simulink model "MultirotorModel"  (R2021b)
settings: Solver=VariableStepAuto  StartTime=0.0  StopTime=200  FixedStep=0.005  RelTol=1e-3  EnableMultiTasking=on
undefined symbols (not defined in the file): Controller, decyear, DiscIntNeverNeededParam, DroneMass, Dz, Earth, Gravity, initialConditions, Iz, leapyear, Nz, Pz, startFlightTime, UAVSampleTime, Vehicle, WGS84
libraries: slpidlib x10, uavalgslib x6, aerolibtransform2 x4, simulink x2, sharedutil x2, aerolibconvert2 x2, aerolibatmos2 x1, aerolibgravity2 x1, shared6dof x1, aerolibasang x1, sensorinslib x1
(part 1 of 3)
settings Model: DataDictionary=uavPackageDeliveryDataDict.sldd  ModifiedByFormat=The MathWorks, Inc.  Creator=The MathWorks, Inc.  LastModifiedBy=The MathWorks, Inc.
settings SolverCC: AlgebraicLoopSolver=TrustRegion  AutoInsertRateTranBlk=on
settings DataIOCC: LimitDataPoints=on  SaveOutput=off  SaveTime=off  ReturnWorkspaceOutputs=off
settings OptimizationCC: LifeSpan=inf
settings DebuggingCC: ParameterPrecisionLossMsg=none  AllowSymbolicDim=off  SFUnexpectedBacktrackingDiag=warning  SFNoUnconditionalDefaultTransitionDiag=warning  SFExecutionAtInitializationDiag=none  SFMachineParentedDataDiag=warning  ArithmeticOperatorsInVariantConditions=warning
settings ModelReferenceCC: PropagateSignalLabelsOutOfModel=off
settings SFSimCC: SimUseLocalCustomCode=off  CustomCodeUndefinedFunction=UseInterfaceOnly
settings RTWCC: RTWUseLocalCustomCode=off
settings CodeAppCC: StateflowObjectComments=on
settings GRTTargetCC: TargetLangStandard=C89/C90 (ANSI)
settings ConfigComp: CovMetricSettings=dw  CovSaveCumulativeToWorkspaceVar=on  CovSaveSingleToWorkspaceVar=on  CovExternalEMLEnable=off

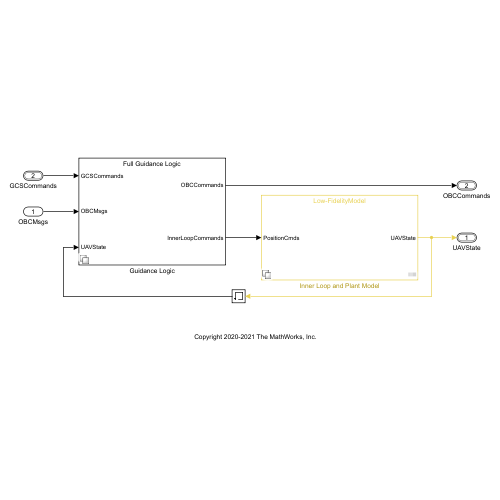
[thumbnail: Simulink's stored preview of the top-level diagram]
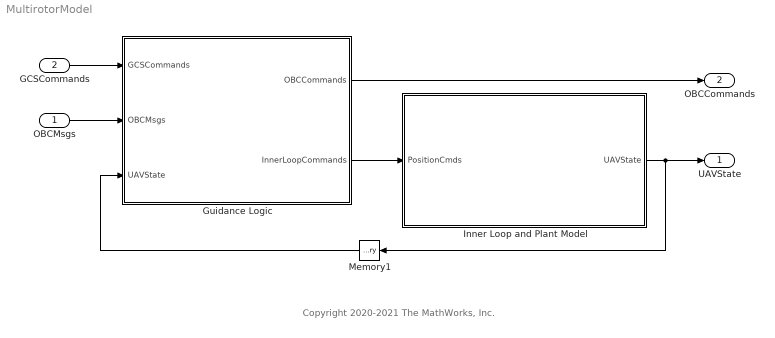
== system MultirotorModel ==
  note: Copyright 2020-2021 The MathWorks, Inc.
  OBCMsgs : Inport  OutDataTypeStr=single  PortDimensions=[1 1]  SampleTime=UAVSampleTime*4
  GCSCommands : Inport  Port=2  OutDataTypeStr=Bus: uavPathManagerBus  PortDimensions=42  SampleTime=UAVSampleTime*4  BusOutputAsStruct=on
  Guidance Logic : Subsystem  Variant=on
  Inner Loop and Plant Model : Subsystem  Variant=on
  Memory1 : Memory  InheritSampleTime=on
  UAVState : Outport  OutDataTypeStr=Bus: uavStateBus  BusOutputAsStruct=on
  OBCCommands : Outport  Port=2  OutDataTypeStr=Bus: uavPathManagerBus  PortDimensions=2  SampleTime=0.005  BusOutputAsStruct=on
  wires:
  GCSCommands/1 -> Guidance Logic/1(GCSCommands)
  OBCMsgs/1 -> Guidance Logic/2(OBCMsgs)
  Guidance Logic/2(InnerLoopCommands) -> Inner Loop and Plant Model/1(PositionCmds)
  Guidance Logic/1(OBCCommands) -> OBCCommands/1
  Inner Loop and Plant Model/1(UAVState) -> Memory1/1, UAVState/1
  Memory1/1 -> Guidance Logic/3(UAVState)

== system MultirotorModel/Guidance Logic ==
  GCSCommands : Inport
  OBCMsgs : Inport  Port=2
  UAVState : Inport  Port=3
  Full Guidance Logic : Subsystem  TreatAsAtomicUnit=on  SystemSampleTime=UAVSampleTime*4  VariantControl=guidanceType==1
  Obstacle Avoidance : Subsystem  TreatAsAtomicUnit=on  SystemSampleTime=0.005*4  VariantControl=guidanceType ==2
  OBCCommands : Outport  SampleTime=0.005  BusOutputAsStruct=on
  InnerLoopCommands : Outport  Port=2

== system MultirotorModel/Inner Loop and Plant Model ==
  PositionCmds : Inport
  High-FidelityModel : Subsystem  VariantControl=plantModelFi==1
  Low-FidelityModel : Subsystem  VariantControl=plantModelFi ==0
  UAVState : Outport

== system MultirotorModel/Guidance Logic/Full Guidance Logic ==
  GCSCommands : Inport
  OBCMsgs : Inport  Port=2
  UAVState : Inport  Port=3
  Atan2 : Trigonometry  Operator=atan2
  Bus Selector1 : BusSelector  OutputSignals=pos_vel.x,pos_vel.y,pos_vel.z,pos_vel.vy,pos_vel.vx
  Ground : Ground
  Guidance Stateflow : Subsystem
  Mux : Mux
  Terminator : Terminator
  InnerLoopCommands : Outport
  OBCCommands : Outport  Port=2  OutDataTypeStr=Bus: uavPathManagerBus  BusOutputAsStruct=on
  wires:
  Mux/1 -> Guidance Stateflow/1(Pose)
  Bus Selector1/5 -> Atan2/2  "<vx>"
  GCSCommands/1 -> Guidance Stateflow/2(GCSCommands)
  Guidance Stateflow/1(InnerLoopCommands) -> InnerLoopCommands/1
  Bus Selector1/4 -> Atan2/1  "<vy>"
  Bus Selector1/3 -> Mux/3  "<z>"
  Bus Selector1/2 -> Mux/2  "<y>"
  UAVState/1 -> Bus Selector1/1
  Atan2/1 -> Mux/4
  Bus Selector1/1 -> Mux/1  "<x>"
  OBCMsgs/1 -> Terminator/1
  Ground/1 -> OBCCommands/1

== system MultirotorModel/Guidance Logic/Obstacle Avoidance ==
  GCSCommands : Inport
  OBCMsgs : Inport  Port=2
  UAVState : Inport  Port=3
  Bus Selector : BusSelector  OutputSignals=pos_vel
  Compute InnerLoop Cmds : Subsystem  TreatAsAtomicUnit=on
  MATLAB Function : MATLAB Function  TreatAsAtomicUnit=on
  Selector : Selector  InputPortWidth=42  IndexOptions=Index vector (dialog)  Indices=[1 2]  OutputSizes=1
  Unit Delay1 : UnitDelay  InitialCondition=single(0)  SampleTime=-1  HasFrameUpgradeWarning=on
  InnerLoopCommands : Outport
  OBCCommands : Outport  Port=2  BusOutputAsStruct=on
  wires:
  OBCMsgs/1 -> Unit Delay1/1
  Selector/1 -> OBCCommands/1, MATLAB Function/1(mission)
  MATLAB Function/1(y) -> Compute InnerLoop Cmds/1(GCSCmds)
  Unit Delay1/1 -> MATLAB Function/2(Steer)
  Bus Selector/1 -> MATLAB Function/3(UAVState)  "<pos_vel>"
  UAVState/1 -> Bus Selector/1, Compute InnerLoop Cmds/3(UAVState)
  Compute InnerLoop Cmds/1(InnerLoopCmds) -> InnerLoopCommands/1
  GCSCommands/1 -> Selector/1
  MATLAB Function/2(DTD) -> Compute InnerLoop Cmds/2(DTD)

== system MultirotorModel/Inner Loop and Plant Model/High-FidelityModel ==
  note: To be replaced with a signal from the GCS to "Start Mission"
  PositionCmds : Inport
  Control System : Subsystem  TreatAsAtomicUnit=on  SystemSampleTime=UAVSampleTime
  Environment : Subsystem  TreatAsAtomicUnit=on  VariantControl=VSS_ENVIRONMENT_VARIABLE
  Memory1 : Memory  InheritSampleTime=on  LinearizeMemory=on  LinearizeAsDelay=on
  Plant Model : Subsystem  TreatAsAtomicUnit=on
  Rate Transition : RateTransition
  Rate Transition1 : RateTransition  OutPortSampleTime=UAVSampleTime
  Rate Transition2 : RateTransition  OutPortSampleTime=UAVSampleTime
  Step : Step  Time=startFlightTime  SampleTime=UAVSampleTime
  UAVState : Outport  OutDataTypeStr=Bus: uavStateBus
  wires:
  PositionCmds/1 -> Rate Transition1/1
  Control System/1(ActuatorCmds) -> Rate Transition/1  "motors"
  Environment/1(Environment) -> Plant Model/2(Environment)
  Memory1/1 -> Environment/1(States), Rate Transition2/1
  Plant Model/1(UAVState) -> UAVState/1, Memory1/1
  Step/1 -> Control System/Enable
  Rate Transition/1 -> Plant Model/1(Actuators)
  Rate Transition1/1 -> Control System/1(PositionCmd)
  Rate Transition2/1 -> Control System/2(UAVState)

== system MultirotorModel/Inner Loop and Plant Model/Low-FidelityModel ==
  PositionCmds : Inport
  Assemble UAV State Bus : Subsystem
  Bus Creator1 : BusCreator  Inputs=1  OutDataTypeStr=Bus: uavGuidanceEnvironmentBus  NonVirtualBus=on
  Constant : Constant  Value=Gravity  OutDataTypeStr=single
      settings: AttributesFormatString=%<Value>
  INS1 : Subsystem
  INS2 : Subsystem
  Position and Acceleration Control : Subsystem
  Quadrotor Plant : uavalgslib/Guidance Model  ModelType=MultirotorGuidance  SpecifiedDataType=single  SimulateUsing=Code generation  InitialWorldPositionMultirotor=[-186; -105; 0]  InitialWorldVelocityMultirotor=[0; 0; 0]  InitialEulerZYXMultirotor=[0; 0; 0]  InitialBodyAngularRateRPYMultirotor=[0; 0; 0]  InitialThrustMultirotor=0  InitialNorthFixedWing=0  InitialEastFixedWing=0  InitialHeightFixedWing=0  InitialAirSpeedFixedWing=0  InitialHeadingAngleFixedWing=0  InitialFlightPathAngleFixedWing=0  InitialRollAngleFixedWing=0  InitialRollAngleRateFixedWing=0  PDRollMultirotor=[3402.97,116.67]  PDPitchMultirotor=[3402.97, 116.67]  PYawRateMultirotor=1950  PThrustMultirotor=39  MassMultirotor=0.1  PHeightFixedWing=3.9  PHeadingAngleFixedWing=3.9  PFlightPathAngleFixedWing=39  PDRollFixedWing=[3402.97, 116.67]  PAirSpeedFixedWing=1  FlightPathAngleLimitsFixedWing=[-pi/2, pi/2]  StateBusName='uavGuidanceStateBus'  ControlBusName='uavGuidanceControlBus'  EnvironmentBusName='uavGuidanceEnvironmentBus'  DataType=single
      settings: SourceProductName=UAV Toolbox
  Rate Transition1 : RateTransition  OutPortSampleTime=UAVSampleTime
  Rate Transition2 : RateTransition  OutPortSampleTime=UAVSampleTime
  UAVState : Outport  OutDataTypeStr=Bus: uavStateBus
  wires:
  Constant/1 -> Bus Creator1/1  "Gravity"
  Bus Creator1/1 -> Quadrotor Plant/2
  Position and Acceleration Control/1(Control Signal) -> Rate Transition2/1
  Quadrotor Plant/1 -> Rate Transition1/1
  Rate Transition2/1 -> Quadrotor Plant/1
  PositionCmds/1 -> Position and Acceleration Control/2(PositionCmd)
  Rate Transition1/1 -> INS2/1(State), INS1/1(State), Assemble UAV State Bus/1(State)
  Assemble UAV State Bus/1(UAVState) -> UAVState/1
  INS1/1(QuadRotorStateGPS) -> Position and Acceleration Control/1(QuadRotorState)
  INS2/1(QuadRotorStateGPS) -> Position and Acceleration Control/3(QuadRotorState1)

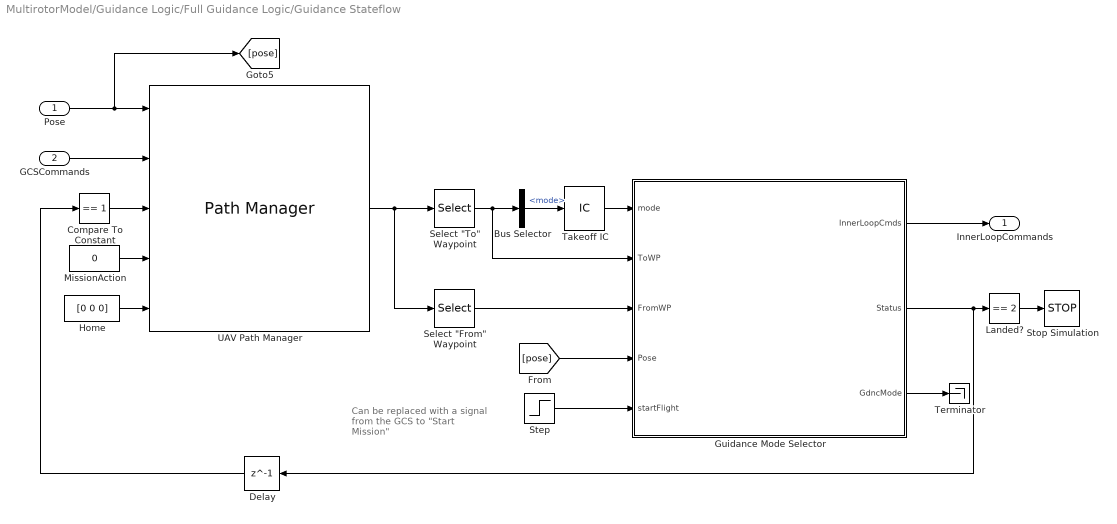
== system MultirotorModel/Guidance Logic/Full Guidance Logic/Guidance Stateflow ==
  note: Can be replaced with a signal from the GCS to "Start Mission"
  Pose : Inport
  GCSCommands : Inport  Port=2
  Bus Selector : BusSelector  OutputSignals=mode
  Compare To Constant : simulink/Logic and Bit Operations/Compare To Constant  relop===  const=1  OutDataTypeStr=boolean
  Delay : Delay  DelayLength=1  InitialCondition=0
  Guidance Mode Selector : Stateflow chart  TreatAsAtomicUnit=on
  Home : Constant  Value=[0 0 0]  OutDataTypeStr=single
  Landed? : simulink/Logic and Bit Operations/Compare To Constant  relop===  const=2  OutDataTypeStr=boolean
  MissionAction : Constant  Value=0  OutDataTypeStr=uint8
  "Select \"From\" Waypoint" : Selector  InputPortWidth=2  IndexOptions=Index vector (dialog)  Indices=2  OutputSizes=1
  "Select \"To\" Waypoint" : Selector  InputPortWidth=2  IndexOptions=Index vector (dialog)  Indices=1  OutputSizes=1
  Step : Step  Time=startFlightTime  SampleTime=UAVSampleTime*4
  Stop Simulation : Stop
  Takeoff IC : InitialCondition
  Terminator : Terminator
  UAV Path Manager : uavalgslib/Path Manager  UAVType=multirotor  LoiterRadius=25  dataType=single  inputBusName='uavPathManagerBus'  SimulateUsing=Code generation
      settings: SourceProductName=UAV Toolbox
  InnerLoopCommands : Outport  OutDataTypeStr=Bus: innerLoopCmdsBus
  wires:
  Takeoff IC/1 -> Guidance Mode Selector/1(mode)
  MissionAction/1 -> UAV Path Manager/4
  Delay/1 -> Compare To Constant/1
  Guidance Mode Selector/2(Status) -> Delay/1, Landed?/1
  Home/1 -> UAV Path Manager/5
  Guidance Mode Selector/1(InnerLoopCmds) -> InnerLoopCommands/1
  GCSCommands/1 -> UAV Path Manager/2
  Pose/1 -> UAV Path Manager/1, [pose]
  UAV Path Manager/1 -> "Select \"From\" Waypoint"/1, "Select \"To\" Waypoint"/1
  Bus Selector/1 -> Takeoff IC/1  "<mode>"
  [pose] -> Guidance Mode Selector/4(Pose)
  Compare To Constant/1 -> UAV Path Manager/3
  "Select \"To\" Waypoint"/1 -> Guidance Mode Selector/2(ToWP), Bus Selector/1
  "Select \"From\" Waypoint"/1 -> Guidance Mode Selector/3(FromWP)
  Landed?/1 -> Stop Simulation/1
  Step/1 -> Guidance Mode Selector/5(startFlight)
  Guidance Mode Selector/3(GdncMode) -> Terminator/1

== system MultirotorModel/Guidance Logic/Obstacle Avoidance/Compute InnerLoop Cmds ==
  GCSCmds : Inport
  DTD : Inport  Port=2
  UAVState : Inport  Port=3
  FollowWaypoints : Subsystem
  GCSCmds1 : InportShadow
  Landing : Subsystem
  Switch1 : Switch  Threshold=5
  UAVState1 : InportShadow  Port=3
  InnerLoopCmds : Outport  OutDataTypeStr=Bus: innerLoopCmdsBus
  wires:
  DTD/1 -> Switch1/2
  UAVState/1 -> FollowWaypoints/1(UAVState)
  GCSCmds/1 -> FollowWaypoints/2(GCSCmds)
  FollowWaypoints/1(InnerLoopCmds) -> Switch1/1
  Switch1/1 -> InnerLoopCmds/1
  UAVState1/1 -> Landing/2(UAVState1)
  GCSCmds1/1 -> Landing/1(GCSCmds)
  Landing/1(InnerLoopCmds1) -> Switch1/3

== system MultirotorModel/Inner Loop and Plant Model/High-FidelityModel/Control System ==
  note: Derived from the work by Sertac
      | Karaman and Fabian Riether
  PositionCmd : Inport
  UAVState : Inport  Port=2  BusOutputAsStruct=on
  Enable : EnablePort  StatesWhenEnabling=reset
  Controller : Subsystem
  ActuatorCmds : Outport  VectorParamsAs1DForOutWhenUnconnected=off
  wires:
  Controller/1(motors_refout) -> ActuatorCmds/1
  UAVState/1 -> Controller/2(UAVState)
  PositionCmd/1 -> Controller/1(PositionCmd)

== system MultirotorModel/Inner Loop and Plant Model/High-FidelityModel/Environment ==
  States : Inport
  Bus Creator : BusCreator  Inputs=3  OutDataTypeStr=Bus: EnvironmentBus  NonVirtualBus=on
  Bus Creator1 : BusCreator  Inputs=4  OutDataTypeStr=Bus: AtmosphereBus  NonVirtualBus=on
  Bus Selector : BusSelector  OutputSignals=gps.lat,gps.lon,gps.alt
  COESA Atmosphere Model : aerolibatmos2/COESA Atmosphere Model  units=Metric (MKS)  spec=1976 COESA-extended U.S. Standard Atmosphere  model=Profile  profile_var=High temperature  profile_percent=1%  profile_alt=5 km (16404 ft)  envelope_var=High temperature  envelope_percent=1%  action=None
  Clock : Clock
  Gain : Gain  Gain=1/1e7  OutDataTypeStr=double
  Gain1 : Gain  Gain=1/1e7  OutDataTypeStr=double
  Gain2 : Gain  Gain=1/-1e3  OutDataTypeStr=double
  Initial date : Constant  Value=decyear(initialConditions.date)
  Mux : Mux  Inputs=3
  Sum : Sum  Inputs=|++
  "WGS84 Gravity Model  " : GravityWGS84  action=None
  World Magnetic Model 2015 : aerolibgravity2/World Magnetic Model  model=WMM2015 V2 (2015-2020)  customFile='WMM2020.COF'  units=Metric (MKS)  time_in=on  month=January  day=1  year=2015  action=Error  h_out=off  dec_out=off  inc_out=off  ti_out=off
      settings: SourceProductBaseCode=AE
  kclock : Gain  Gain=1/(60*60*24*(365 + leapyear(initialConditions.date(1))))
  Environment : Outport  VectorParamsAs1DForOutWhenUnconnected=off
  wires:
  States/1 -> Bus Selector/1  "StatesLog"
  Bus Creator/1 -> Environment/1
  COESA Atmosphere Model/1 -> Bus Creator1/1  "air_temp"
  COESA Atmosphere Model/2 -> Bus Creator1/2  "speed_sound"
  COESA Atmosphere Model/3 -> Bus Creator1/3  "pressure"
  COESA Atmosphere Model/4 -> Bus Creator1/4  "air_density"
  Bus Creator1/1 -> Bus Creator/2  "AtmosphereBus"
  World Magnetic Model 2015/1 -> Bus Creator/3  "MagneticField_ned"
  "WGS84 Gravity Model  "/1 -> Bus Creator/1  "Gravity_ned"
  Clock/1 -> kclock/1
  Initial date/1 -> Sum/1
  Sum/1 -> World Magnetic Model 2015/4
  kclock/1 -> Sum/2
  Mux/1 -> "WGS84 Gravity Model  "/1
  Gain/1 -> World Magnetic Model 2015/2, Mux/1
  Bus Selector/1 -> Gain/1  "<lat>"
  Bus Selector/2 -> Gain1/1  "<lon>"
  Gain1/1 -> World Magnetic Model 2015/3, Mux/2
  Bus Selector/3 -> Gain2/1  "<alt>"
  Gain2/1 -> COESA Atmosphere Model/1, World Magnetic Model 2015/1, Mux/3

== system MultirotorModel/Inner Loop and Plant Model/High-FidelityModel/Plant Model ==
  Actuators : Inport
  Environment : Inport  Port=2
  6DOF (Quaternion) : shared6dof/6DOF (Euler Angles)  units=Metric (MKS)  mtype=Fixed  rep=Euler Angles  xme_0=initialConditions.posNED + [0 0 -1]  Vm_0=[0 0 0]  eul_0=[0,0,0]  pm_0=[0,0,0]  mass_0=Vehicle.Airframe.mass  mass_e=0.5  mass_f=2.0  inertia=Vehicle.Airframe.inertia  inertia_e=eye(3)  inertia_f=2*eye(3)  k_quat=Vehicle.SixDOF.quatGain  vre_flag=on  abi_flag=on  aMode=aMode  xme_statename=''  Vm_statename=''  eul_statename=''  quat_statename=''  pm_statename=''  mass_statename=''
      settings: SourceProductBaseCode=AE,PW,DR,MT,UV,VE
  AC model : Subsystem
  Bus setup : Subsystem
  Terminator1 : Terminator
  Terminator2 : Terminator
  Terminator3 : Terminator
  UAVState : Outport  VectorParamsAs1DForOutWhenUnconnected=off
  wires:
  Actuators/1 -> AC model/1(Actuators)
  Environment/1 -> AC model/2(Environment)
  AC model/1(F_cg) -> 6DOF (Quaternion)/1
  AC model/2(M_cg) -> 6DOF (Quaternion)/2
  6DOF (Quaternion)/1 -> Bus setup/1(V_ned)
  6DOF (Quaternion)/2 -> Bus setup/2(X_ned)
  6DOF (Quaternion)/3 -> Bus setup/3(Euler)
  6DOF (Quaternion)/6 -> Bus setup/5(Omega_b), AC model/5(w_b)
  6DOF (Quaternion)/5 -> AC model/4(V_b)
  6DOF (Quaternion)/4 -> Bus setup/4(DCM), AC model/3(DCM_be)
  Bus setup/1(UAVState) -> UAVState/1
  6DOF (Quaternion)/9 -> Terminator1/1
  6DOF (Quaternion)/7 -> Terminator2/1
  6DOF (Quaternion)/8 -> Terminator3/1

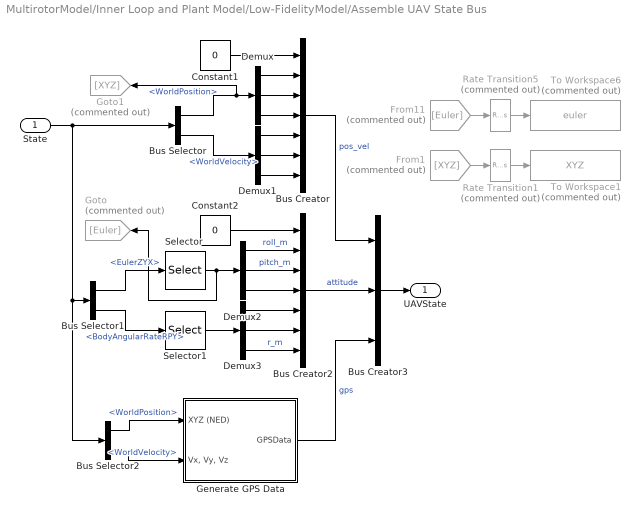
== system MultirotorModel/Inner Loop and Plant Model/Low-FidelityModel/Assemble UAV State Bus ==
  State : Inport
  Bus Creator : BusCreator  Inputs=7  OutDataTypeStr=Bus: local_position_ned
      settings: InheritFromInputs=off
  Bus Creator2 : BusCreator  Inputs=7  OutDataTypeStr=Bus: attitudeBus
      settings: InheritFromInputs=off
  Bus Creator3 : BusCreator  Inputs=3  OutDataTypeStr=Bus: uavStateBus
      settings: InheritFromInputs=off
  Bus Selector : BusSelector  OutputSignals=WorldPosition,WorldVelocity
  Bus Selector1 : BusSelector  OutputSignals=EulerZYX,BodyAngularRateRPY
  Bus Selector2 : BusSelector  OutputSignals=WorldPosition,WorldVelocity
  Constant1 : Constant  Value=0  OutDataTypeStr=uint32
  Constant2 : Constant  Value=0  OutDataTypeStr=uint32
  Demux{,1..3} (4 alike) : Demux  Outputs=3
  From1 : From  Commented=on  GotoTag=XYZ
  From11 : From  Commented=on  GotoTag=Euler
  Generate GPS Data : Subsystem
  Goto : Goto  Commented=on  GotoTag=Euler
  Goto1 : Goto  Commented=on  GotoTag=XYZ
  Rate Transition1 : RateTransition  Commented=on  OutPortSampleTime=UAVSampleTime
  Rate Transition5 : RateTransition  Commented=on  OutPortSampleTime=UAVSampleTime
  Selector : Selector  InputPortWidth=3  IndexOptions=Index vector (dialog)  Indices=[3 2 1]  OutputSizes=1
  Selector1 : Selector  InputPortWidth=3  IndexOptions=Index vector (dialog)  Indices=[3 2 1]  OutputSizes=1
  To Workspace1 : ToWorkspace  Commented=on  VariableName=XYZ  SaveFormat=Timeseries  SampleTime=-1
  To Workspace6 : ToWorkspace  Commented=on  VariableName=euler  SaveFormat=Timeseries  SampleTime=-1
  UAVState : Outport  OutDataTypeStr=Bus: uavStateBus
  wires:
  Bus Creator2/1 -> Bus Creator3/2  "attitude"
  Bus Creator3/1 -> UAVState/1
  Demux3/1 -> Bus Creator2/5
  Demux1/2 -> Bus Creator/6
  Bus Creator/1 -> Bus Creator3/1  "pos_vel"
  Demux1/3 -> Bus Creator/7
  Bus Selector2/2 -> Generate GPS Data/2("Vx, Vy, Vz")  "<WorldVelocity>"
  Demux/1 -> Bus Creator/2
  State/1 -> Bus Selector/1, Bus Selector2/1, Bus Selector1/1
  Constant2/1 -> Bus Creator2/1
  Bus Selector/1 -> Goto1/1, Demux/1  "<WorldPosition>"
  Selector1/1 -> Demux3/1
  Demux1/1 -> Bus Creator/5
  Bus Selector1/1 -> Selector/1  "<EulerZYX>"
  Demux/2 -> Bus Creator/3
  Demux2/1 -> Bus Creator2/2  "roll_m"
  Demux2/3 -> Bus Creator2/4
  Demux3/2 -> Bus Creator2/6
  Demux2/2 -> Bus Creator2/3  "pitch_m"
  Bus Selector1/2 -> Selector1/1  "<BodyAngularRateRPY>"
  Demux3/3 -> Bus Creator2/7  "r_m"
  Demux/3 -> Bus Creator/4
  Bus Selector/2 -> Demux1/1  "<WorldVelocity>"
  Constant1/1 -> Bus Creator/1
  Bus Selector2/1 -> Generate GPS Data/1(XYZ (NED))  "<WorldPosition>"
  Generate GPS Data/1(GPSData) -> Bus Creator3/3  "gps"
  Rate Transition5/1 -> To Workspace6/1
  From11/1 -> Rate Transition5/1
  Selector/1 -> Goto/1, Demux2/1
  From1/1 -> Rate Transition1/1
  Rate Transition1/1 -> To Workspace1/1

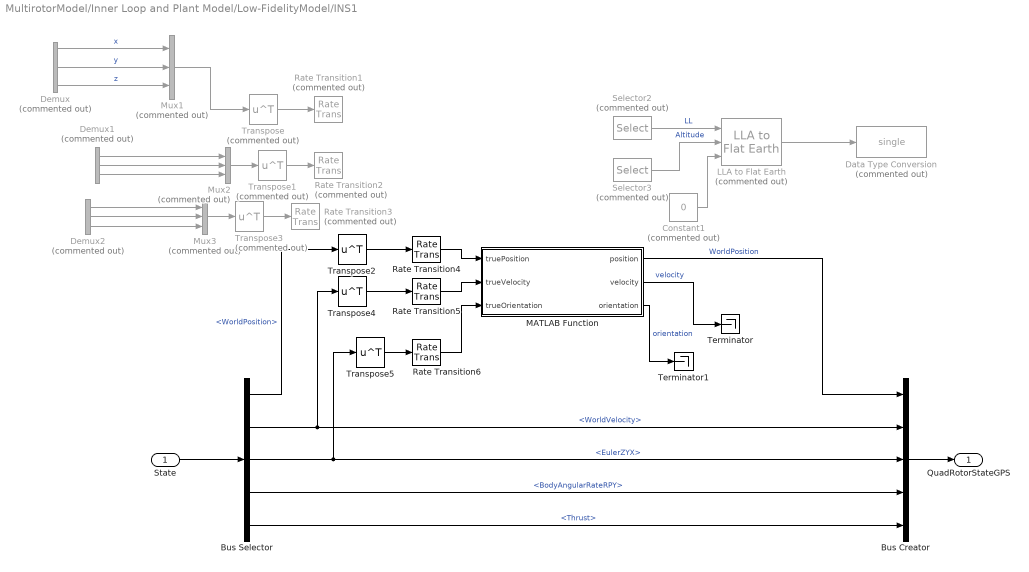
== system MultirotorModel/Inner Loop and Plant Model/Low-FidelityModel/INS1 ==
  State : Inport
  Bus Creator : BusCreator  Inputs=5
  Bus Selector : BusSelector  OutputSignals=WorldPosition,WorldVelocity,EulerZYX,BodyAngularRateRPY,Thrust
  Constant1 : Constant  Commented=on  Value=0
  Data Type Conversion : DataTypeConversion  Commented=on  OutDataTypeStr=single
  Demux : Demux  Commented=on  Outputs=3
  Demux1 : Demux  Commented=on  Outputs=3
  Demux2 : Demux  Commented=on  Outputs=3
  LLA to Flat Earth : aerolibtransform2/LLA to Flat Earth  Commented=on  units=Metric (MKS)  ptype=Earth (WGS84)  F=1/298.257223563  R=6378137  refPosPort=off  LL0=[41.8856528 -87.6556726]  psi=0
      settings: SourceProductBaseCode=AE
  MATLAB Function : MATLAB Function  TreatAsAtomicUnit=on
  Mux1 : Mux  Commented=on  Inputs=3
  Mux2 : Mux  Commented=on  Inputs=3
  Mux3 : Mux  Commented=on  Inputs=3
  Rate Transition1 : RateTransition  Commented=on  OutPortSampleTime=UAVSampleTime
  Rate Transition2 : RateTransition  Commented=on  OutPortSampleTime=UAVSampleTime
  Rate Transition3 : RateTransition  Commented=on  OutPortSampleTime=UAVSampleTime
  Rate Transition4 : RateTransition  OutPortSampleTime=UAVSampleTime
  Rate Transition5 : RateTransition  OutPortSampleTime=UAVSampleTime
  Rate Transition6 : RateTransition  OutPortSampleTime=UAVSampleTime
  Selector2 : Selector  Commented=on  InputPortWidth=3  IndexOptions=Index vector (dialog)  Indices=[1 2]  OutputSizes=1
  Selector3 : Selector  Commented=on  InputPortWidth=3  IndexOptions=Index vector (dialog)  Indices=[3]  OutputSizes=1
  Terminator : Terminator
  Terminator1 : Terminator
  Transpose : Math  Commented=on  Operator=transpose  SaturateOnIntegerOverflow=on
  Transpose1 : Math  Commented=on  Operator=transpose  SaturateOnIntegerOverflow=on
  Transpose2 : Math  Operator=transpose  SaturateOnIntegerOverflow=on
  Transpose3 : Math  Commented=on  Operator=transpose  SaturateOnIntegerOverflow=on
  Transpose4 : Math  Operator=transpose  SaturateOnIntegerOverflow=on
  Transpose5 : Math  Operator=transpose  SaturateOnIntegerOverflow=on
  QuadRotorStateGPS : Outport
  wires:
  State/1 -> Bus Selector/1
  Bus Creator/1 -> QuadRotorStateGPS/1
  Bus Selector/2 -> Transpose4/1, Bus Creator/2  "<WorldVelocity>"
  Bus Selector/3 -> Bus Creator/3, Transpose5/1  "<EulerZYX>"
  Bus Selector/4 -> Bus Creator/4  "<BodyAngularRateRPY>"
  Bus Selector/5 -> Bus Creator/5  "<Thrust>"
  Demux/1 -> Mux1/1  "x"
  Transpose/1 -> Rate Transition1/1
  Selector3/1 -> LLA to Flat Earth/2  "Altitude"
  Selector2/1 -> LLA to Flat Earth/1  "LL"
  MATLAB Function/3(orientation) -> Terminator1/1  "orientation"
  Mux2/1 -> Transpose1/1
  Mux1/1 -> Transpose/1
  Constant1/1 -> LLA to Flat Earth/3
  LLA to Flat Earth/1 -> Data Type Conversion/1
  Transpose1/1 -> Rate Transition2/1
  MATLAB Function/2(velocity) -> Terminator/1  "velocity"
  Mux3/1 -> Transpose3/1
  Transpose3/1 -> Rate Transition3/1
  Demux2/3 -> Mux3/3
  Demux/2 -> Mux1/2  "y"
  Demux/3 -> Mux1/3  "z"
  Demux1/1 -> Mux2/1
  Demux1/2 -> Mux2/2
  Demux1/3 -> Mux2/3
  Demux2/1 -> Mux3/1
  Demux2/2 -> Mux3/2
  Bus Selector/1 -> Transpose2/1  "<WorldPosition>"
  Transpose2/1 -> Rate Transition4/1
  Rate Transition4/1 -> MATLAB Function/1(truePosition)
  Transpose4/1 -> Rate Transition5/1
  Rate Transition5/1 -> MATLAB Function/2(trueVelocity)
  Transpose5/1 -> Rate Transition6/1
  Rate Transition6/1 -> MATLAB Function/3(trueOrientation)
  MATLAB Function/1(position) -> Bus Creator/1  "WorldPosition"

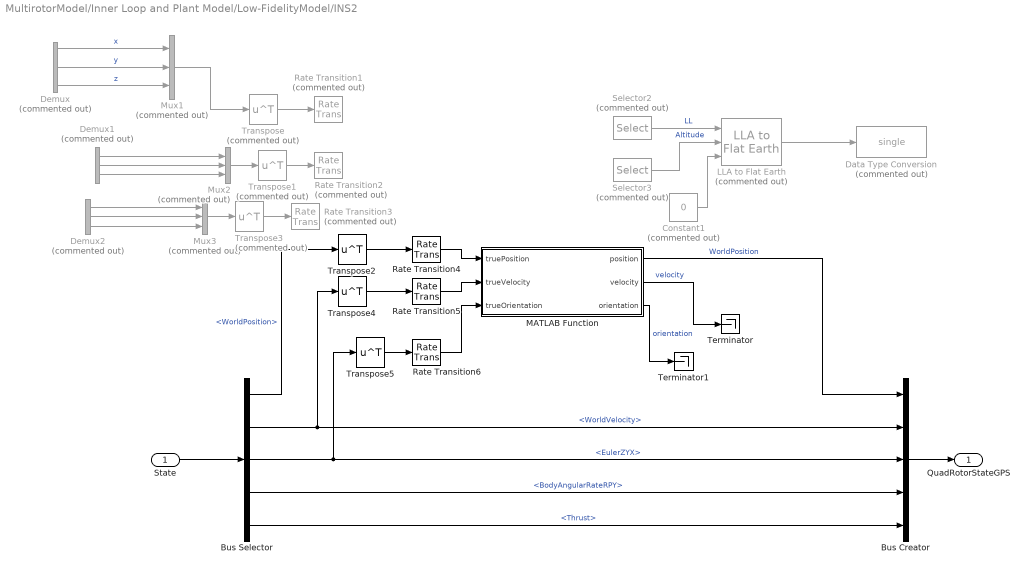
== system MultirotorModel/Inner Loop and Plant Model/Low-FidelityModel/INS2 ==
  State : Inport
  Bus Creator : BusCreator  Inputs=5
  Bus Selector : BusSelector  OutputSignals=WorldPosition,WorldVelocity,EulerZYX,BodyAngularRateRPY,Thrust
  Constant1 : Constant  Commented=on  Value=0
  Data Type Conversion : DataTypeConversion  Commented=on  OutDataTypeStr=single
  Demux : Demux  Commented=on  Outputs=3
  Demux1 : Demux  Commented=on  Outputs=3
  Demux2 : Demux  Commented=on  Outputs=3
  LLA to Flat Earth : aerolibtransform2/LLA to Flat Earth  Commented=on  units=Metric (MKS)  ptype=Earth (WGS84)  F=1/298.257223563  R=6378137  refPosPort=off  LL0=[41.8856528 -87.6556726]  psi=0
      settings: SourceProductBaseCode=AE
  MATLAB Function : MATLAB Function  TreatAsAtomicUnit=on
  Mux1 : Mux  Commented=on  Inputs=3
  Mux2 : Mux  Commented=on  Inputs=3
  Mux3 : Mux  Commented=on  Inputs=3
  Rate Transition1 : RateTransition  Commented=on  OutPortSampleTime=UAVSampleTime
  Rate Transition2 : RateTransition  Commented=on  OutPortSampleTime=UAVSampleTime
  Rate Transition3 : RateTransition  Commented=on  OutPortSampleTime=UAVSampleTime
  Rate Transition4 : RateTransition  OutPortSampleTime=UAVSampleTime
  Rate Transition5 : RateTransition  OutPortSampleTime=UAVSampleTime
  Rate Transition6 : RateTransition  OutPortSampleTime=UAVSampleTime
  Selector2 : Selector  Commented=on  InputPortWidth=3  IndexOptions=Index vector (dialog)  Indices=[1 2]  OutputSizes=1
  Selector3 : Selector  Commented=on  InputPortWidth=3  IndexOptions=Index vector (dialog)  Indices=[3]  OutputSizes=1
  Terminator : Terminator
  Terminator1 : Terminator
  Transpose : Math  Commented=on  Operator=transpose  SaturateOnIntegerOverflow=on
  Transpose1 : Math  Commented=on  Operator=transpose  SaturateOnIntegerOverflow=on
  Transpose2 : Math  Operator=transpose  SaturateOnIntegerOverflow=on
  Transpose3 : Math  Commented=on  Operator=transpose  SaturateOnIntegerOverflow=on
  Transpose4 : Math  Operator=transpose  SaturateOnIntegerOverflow=on
  Transpose5 : Math  Operator=transpose  SaturateOnIntegerOverflow=on
  QuadRotorStateGPS : Outport
  wires:
  State/1 -> Bus Selector/1
  Bus Creator/1 -> QuadRotorStateGPS/1
  Bus Selector/2 -> Transpose4/1, Bus Creator/2  "<WorldVelocity>"
  Bus Selector/3 -> Bus Creator/3, Transpose5/1  "<EulerZYX>"
  Bus Selector/4 -> Bus Creator/4  "<BodyAngularRateRPY>"
  Bus Selector/5 -> Bus Creator/5  "<Thrust>"
  Demux/1 -> Mux1/1  "x"
  Transpose/1 -> Rate Transition1/1
  Selector3/1 -> LLA to Flat Earth/2  "Altitude"
  Selector2/1 -> LLA to Flat Earth/1  "LL"
  MATLAB Function/3(orientation) -> Terminator1/1  "orientation"
  Mux2/1 -> Transpose1/1
  Mux1/1 -> Transpose/1
  Constant1/1 -> LLA to Flat Earth/3
  LLA to Flat Earth/1 -> Data Type Conversion/1
  Transpose1/1 -> Rate Transition2/1
  MATLAB Function/2(velocity) -> Terminator/1  "velocity"
  Mux3/1 -> Transpose3/1
  Transpose3/1 -> Rate Transition3/1
  Demux2/3 -> Mux3/3
  Demux/2 -> Mux1/2  "y"
  Demux/3 -> Mux1/3  "z"
  Demux1/1 -> Mux2/1
  Demux1/2 -> Mux2/2
  Demux1/3 -> Mux2/3
  Demux2/1 -> Mux3/1
  Demux2/2 -> Mux3/2
  Bus Selector/1 -> Transpose2/1  "<WorldPosition>"
  Transpose2/1 -> Rate Transition4/1
  Rate Transition4/1 -> MATLAB Function/1(truePosition)
  Transpose4/1 -> Rate Transition5/1
  Rate Transition5/1 -> MATLAB Function/2(trueVelocity)
  Transpose5/1 -> Rate Transition6/1
  Rate Transition6/1 -> MATLAB Function/3(trueOrientation)
  MATLAB Function/1(position) -> Bus Creator/1  "WorldPosition"

== system MultirotorModel/Inner Loop and Plant Model/Low-FidelityModel/Position and Acceleration Control ==
  note: To be replaced with a signal from the GCS to "Start Mission"
  QuadRotorState : Inport
  PositionCmd : Inport  Port=2
  QuadRotorState1 : Inport  Port=3
  Attitude Control : Subsystem
  Position Control : Subsystem
  Step : Step  Time=startFlightTime  SampleTime=UAVSampleTime
  Velocity Control : Subsystem
  Control Signal : Outport
  wires:
  PositionCmd/1 -> Position Control/1(PositionCmd), Attitude Control/3(PositionCmd)
  Velocity Control/1(Accel Cmd) -> Attitude Control/1(Accel Cmd)
  Attitude Control/1(Control Signal) -> Control Signal/1
  QuadRotorState/1 -> Velocity Control/2(QuadRotorState), Attitude Control/2(QuadRotorState), Position Control/2(QuadRotorState)
  Position Control/1(Velocity Cmd) -> Velocity Control/1(Velocity Cmd)
  Step/1 -> Velocity Control/Enable, Position Control/Enable
  QuadRotorState1/1 -> Position Control/3(QuadRotorState1)

== system MultirotorModel/Guidance Logic/Full Guidance Logic/Guidance Stateflow/Guidance Mode Selector/GuidanceLogic.Land.Descend ==
  ToWP : Inport
  Action Port : ActionPort
      settings: CopyFcn=Stateflow.SLINSF.SimulinkMan.removeBlockPreDeleteFcn  PreDeleteFcn=Stateflow.SLINSF.SimulinkMan.unsafePredeleteFcn
  Bus Creator : BusCreator  Inputs=3  OutDataTypeStr=Bus: innerLoopCmdsBus  NonVirtualBus=on
      settings: InheritFromInputs=off
  Bus Selector : BusSelector  OutputSignals=position,params
  Demux1 : Demux  Outputs=[2 1]
  Hdg Cmd Sat : Saturate  UpperLimit=pi  LowerLimit=-pi
      settings: AttributesFormatString=[%<UpperLimit> %<LowerLimit>]
  Mux : Mux  Inputs=2
  Selector1 : Selector  InputPortWidth=4  IndexOptions=Index vector (dialog)  Indices=4  OutputSizes=1
  Selector3 : Selector  InputPortWidth=4  IndexOptions=Index vector (dialog)  Indices=4  OutputSizes=1
  Yaw Cmd Sat : Saturate  UpperLimit=pi  LowerLimit=-pi
      settings: AttributesFormatString=[%<UpperLimit> %<LowerLimit>]
  InnerLoopCmds : Outport  OutDataTypeStr=Bus: innerLoopCmdsBus
  wires:
  Bus Creator/1 -> InnerLoopCmds/1
  Mux/1 -> Bus Creator/1  "LAP"
  Bus Selector/2 -> Selector1/1, Selector3/1  "<params>"
  Bus Selector/1 -> Demux1/1  "<position>"
  Yaw Cmd Sat/1 -> Bus Creator/3  "YawCmd"
  Hdg Cmd Sat/1 -> Bus Creator/2  "HeadingCmd"
  ToWP/1 -> Bus Selector/1
  Demux1/2 -> Mux/2
  Demux1/1 -> Mux/1
  Selector1/1 -> Yaw Cmd Sat/1
  Selector3/1 -> Hdg Cmd Sat/1

== system MultirotorModel/Guidance Logic/Full Guidance Logic/Guidance Stateflow/Guidance Mode Selector/GuidanceLogic.Land.ToLand ==
  Pose : Inport
  ToWP : Inport  Port=2
  FromWP : Inport  Port=3
  Action Port : ActionPort
      settings: CopyFcn=Stateflow.SLINSF.SimulinkMan.removeBlockPreDeleteFcn  PreDeleteFcn=Stateflow.SLINSF.SimulinkMan.unsafePredeleteFcn
  Bus Creator1 : BusCreator  Inputs=3  OutDataTypeStr=Bus: innerLoopCmdsBus  NonVirtualBus=on
  Constant : Constant  Value=0  OutDataTypeStr=uint8
  Lookahead Distance : Constant  Value=15  OutDataTypeStr=single
  MATLAB Function : MATLAB Function  TreatAsAtomicUnit=on
  Scope : Scope
  Waypoint Follower : uavalgslib/Waypoint Follower  UAVType=multirotor  StartFrom=closest  TransitionRadiusSource=internal  TransitionRadius=10  MinLookaheadDistance=0.1  YawInput=on  ShowCrossTrackErrorOutput=off  ShowStatusOutput=off  SimulateUsing=Code generation
      settings: SourceProductName=UAV Toolbox
  Status : Outport
  InnerLoopCmds : Outport  Port=2  OutDataTypeStr=Bus: innerLoopCmdsBus
  wires:
  Constant/1 -> Status/1
  MATLAB Function/1(wps) -> Waypoint Follower/2
  Lookahead Distance/1 -> Waypoint Follower/3
  Waypoint Follower/1 -> Bus Creator1/1  "LAP"
  Bus Creator1/1 -> InnerLoopCmds/1
  ToWP/1 -> MATLAB Function/2(ToWP)
  Waypoint Follower/2 -> Bus Creator1/2  "HeadingCmd"
  FromWP/1 -> MATLAB Function/1(FromWP)
  Waypoint Follower/4 -> Scope/1
  Waypoint Follower/3 -> Bus Creator1/3  "YawCmd"
  Pose/1 -> Waypoint Follower/1

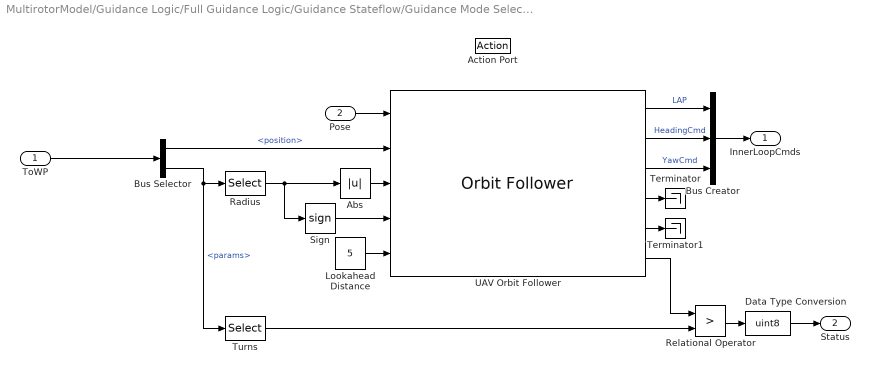
== system MultirotorModel/Guidance Logic/Full Guidance Logic/Guidance Stateflow/Guidance Mode Selector/GuidanceLogic.Orbit ==
  ToWP : Inport
  Pose : Inport  Port=2
  Action Port : ActionPort
      settings: CopyFcn=Stateflow.SLINSF.SimulinkMan.removeBlockPreDeleteFcn  PreDeleteFcn=Stateflow.SLINSF.SimulinkMan.unsafePredeleteFcn
  Abs : Abs
  Bus Creator : BusCreator  Inputs=3  OutDataTypeStr=Bus: innerLoopCmdsBus  NonVirtualBus=on
  Bus Selector : BusSelector  OutputSignals=position,params
  Data Type Conversion : DataTypeConversion  OutDataTypeStr=uint8
  Lookahead Distance : Constant  Value=5  OutDataTypeStr=single
  Radius : Selector  InputPortWidth=4  IndexOptions=Index vector (dialog)  Indices=[3]  OutputSizes=1
  Relational Operator : RelationalOperator  Operator=>  OutDataTypeStr=boolean  RndMeth=Simplest
  Sign : Signum  ZeroCross=off
  Terminator : Terminator
  Terminator1 : Terminator
  Turns : Selector  InputPortWidth=4  IndexOptions=Index vector (dialog)  Indices=[1]  OutputSizes=1
  UAV Orbit Follower : uavalgslib/Orbit Follower  UAVType=multirotor  MinOrbitRadius=1  MinLookaheadDistance=0.1  ExternalReset=none  ShowCrossTrackErrorOutput=off  ShowNumTurnsOutput=on  SimulateUsing=Code generation
      settings: SourceProductName=UAV Toolbox
  InnerLoopCmds : Outport  OutDataTypeStr=Bus: innerLoopCmdsBus
  Status : Outport  Port=2
  wires:
  Pose/1 -> UAV Orbit Follower/1
  Lookahead Distance/1 -> UAV Orbit Follower/5
  Abs/1 -> UAV Orbit Follower/3
  Bus Selector/1 -> UAV Orbit Follower/2  "<position>"
  ToWP/1 -> Bus Selector/1
  UAV Orbit Follower/1 -> Bus Creator/1  "LAP"
  Bus Creator/1 -> InnerLoopCmds/1
  UAV Orbit Follower/2 -> Bus Creator/2  "HeadingCmd"
  UAV Orbit Follower/3 -> Bus Creator/3  "YawCmd"
  Bus Selector/2 -> Turns/1, Radius/1  "<params>"
  Radius/1 -> Abs/1, Sign/1
  Sign/1 -> UAV Orbit Follower/4
  Relational Operator/1 -> Data Type Conversion/1
  Turns/1 -> Relational Operator/2
  Data Type Conversion/1 -> Status/1
  UAV Orbit Follower/6 -> Relational Operator/1
  UAV Orbit Follower/4 -> Terminator/1
  UAV Orbit Follower/5 -> Terminator1/1

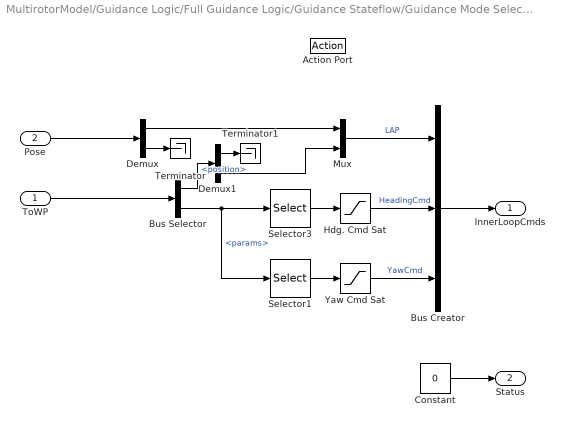
== system MultirotorModel/Guidance Logic/Full Guidance Logic/Guidance Stateflow/Guidance Mode Selector/GuidanceLogic.Takeoff ==
  ToWP : Inport
  Pose : Inport  Port=2
  Action Port : ActionPort
      settings: CopyFcn=Stateflow.SLINSF.SimulinkMan.removeBlockPreDeleteFcn  PreDeleteFcn=Stateflow.SLINSF.SimulinkMan.unsafePredeleteFcn
  Bus Creator : BusCreator  Inputs=3  OutDataTypeStr=Bus: innerLoopCmdsBus  NonVirtualBus=on
      settings: InheritFromInputs=off
  Bus Selector : BusSelector  OutputSignals=position,params
  Constant : Constant  Value=0  OutDataTypeStr=uint8
  Demux : Demux  Outputs=[2 2]
  Demux1 : Demux  Outputs=[2 1]
  Hdg. Cmd Sat : Saturate  UpperLimit=pi  LowerLimit=-pi
      settings: AttributesFormatString=[%<UpperLimit> %<LowerLimit>]
  Mux : Mux  Inputs=2
  Selector1 : Selector  InputPortWidth=4  IndexOptions=Index vector (dialog)  Indices=4  OutputSizes=1
  Selector3 : Selector  InputPortWidth=4  IndexOptions=Index vector (dialog)  Indices=4  OutputSizes=1
  Terminator : Terminator
  Terminator1 : Terminator
  Yaw Cmd Sat : Saturate  UpperLimit=pi  LowerLimit=-pi
      settings: AttributesFormatString=[%<UpperLimit> %<LowerLimit>]
  InnerLoopCmds : Outport  OutDataTypeStr=Bus: innerLoopCmdsBus
  Status : Outport  Port=2
  wires:
  Hdg. Cmd Sat/1 -> Bus Creator/2  "HeadingCmd"
  Bus Creator/1 -> InnerLoopCmds/1
  Constant/1 -> Status/1
  Pose/1 -> Demux/1
  Yaw Cmd Sat/1 -> Bus Creator/3  "YawCmd"
  ToWP/1 -> Bus Selector/1
  Bus Selector/2 -> Selector1/1, Selector3/1  "<params>"
  Mux/1 -> Bus Creator/1  "LAP"
  Demux/1 -> Mux/1
  Bus Selector/1 -> Demux1/1  "<position>"
  Demux1/2 -> Mux/2
  Demux/2 -> Terminator/1
  Demux1/1 -> Terminator1/1
  Selector3/1 -> Hdg. Cmd Sat/1
  Selector1/1 -> Yaw Cmd Sat/1

== system MultirotorModel/Guidance Logic/Full Guidance Logic/Guidance Stateflow/Guidance Mode Selector/GuidanceLogic.WP ==
  FromWP : Inport
  Pose : Inport  Port=2
  ToWP : Inport  Port=3
  Action Port : ActionPort
      settings: CopyFcn=Stateflow.SLINSF.SimulinkMan.removeBlockPreDeleteFcn  PreDeleteFcn=Stateflow.SLINSF.SimulinkMan.unsafePredeleteFcn
  Bus Creator : BusCreator  Inputs=3  OutDataTypeStr=Bus: innerLoopCmdsBus  NonVirtualBus=on
  Data Type Conversion : DataTypeConversion  OutDataTypeStr=uint8
  Dist2WP : Subsystem
  Lookahead Distance : Constant  Value=15  OutDataTypeStr=single
  MATLAB Function : MATLAB Function  TreatAsAtomicUnit=on
  Relational Operator : RelationalOperator  OutDataTypeStr=boolean  RndMeth=Simplest
  Scope : Scope
  Waypoint Follower : uavalgslib/Waypoint Follower  UAVType=multirotor  StartFrom=closest  TransitionRadiusSource=internal  TransitionRadius=10  MinLookaheadDistance=0.1  YawInput=on  ShowCrossTrackErrorOutput=off  ShowStatusOutput=off  SimulateUsing=Code generation
      settings: SourceProductName=UAV Toolbox
  InnerLoopCmds : Outport  OutDataTypeStr=Bus: innerLoopCmdsBus
  Status : Outport  Port=2
  wires:
  Data Type Conversion/1 -> Status/1
  Bus Creator/1 -> InnerLoopCmds/1
  ToWP/1 -> Dist2WP/3(ToWP), MATLAB Function/2(ToWP)
  Waypoint Follower/1 -> Bus Creator/1  "LAP"
  MATLAB Function/1(wps) -> Waypoint Follower/2
  Waypoint Follower/2 -> Bus Creator/2  "HeadingCmd"
  Waypoint Follower/3 -> Bus Creator/3  "YawCmd"
  Lookahead Distance/1 -> Relational Operator/1, Waypoint Follower/3
  Pose/1 -> Waypoint Follower/1, Dist2WP/1(Pose)
  Waypoint Follower/4 -> Scope/1
  Dist2WP/1(Dist) -> Relational Operator/2
  FromWP/1 -> Dist2WP/2(FromWP), MATLAB Function/1(FromWP)
  Relational Operator/1 -> Data Type Conversion/1

== system MultirotorModel/Guidance Logic/Obstacle Avoidance/Compute InnerLoop Cmds/FollowWaypoints ==
  UAVState : Inport
  GCSCmds : Inport  Port=2
  Atan2 : Trigonometry  Operator=atan2
  Bus Creator : BusCreator  Inputs=3  OutDataTypeStr=Bus: innerLoopCmdsBus  NonVirtualBus=on
  Bus Selector1 : BusSelector  OutputSignals=pos_vel.x,pos_vel.y,pos_vel.z,pos_vel.vy,pos_vel.vx
  Lookahead Distance : Constant  Value=5  OutDataTypeStr=single
  Mux : Mux
  Scope : Scope
  Scope1 : Scope
  Terminator : Terminator
  Waypoint Follower : uavalgslib/Waypoint Follower  UAVType=multirotor  StartFrom=first  TransitionRadiusSource=internal  TransitionRadius=0.5  MinLookaheadDistance=0.1  YawInput=on  ShowCrossTrackErrorOutput=on  ShowStatusOutput=on  SimulateUsing=Code generation
      settings: SourceProductName=UAV Toolbox
  InnerLoopCmds : Outport  OutDataTypeStr=Bus: innerLoopCmdsBus
  wires:
  Bus Creator/1 -> InnerLoopCmds/1
  Bus Selector1/4 -> Atan2/1  "<vy>"
  Mux/1 -> Waypoint Follower/1
  Bus Selector1/2 -> Mux/2  "<y>"
  Waypoint Follower/6 -> Scope1/1
  Bus Selector1/3 -> Mux/3  "<z>"
  Bus Selector1/1 -> Mux/1  "<x>"
  Bus Selector1/5 -> Atan2/2  "<vx>"
  Waypoint Follower/2 -> Bus Creator/2  "HeadingCmd"
  Waypoint Follower/3 -> Bus Creator/3  "YawCmd"
  Waypoint Follower/5 -> Scope/1
  Lookahead Distance/1 -> Waypoint Follower/3
  Waypoint Follower/4 -> Terminator/1
  Atan2/1 -> Mux/4
  GCSCmds/1 -> Waypoint Follower/2
  Waypoint Follower/1 -> Bus Creator/1  "LAP"
  UAVState/1 -> Bus Selector1/1

== system MultirotorModel/Guidance Logic/Obstacle Avoidance/Compute InnerLoop Cmds/Landing ==
  GCSCmds : Inport
  UAVState1 : Inport  Port=2  OutDataTypeStr=Bus: uavStateBus
  Atan1 : Trigonometry  Operator=atan2
  Bus Creator1 : BusCreator  Inputs=3  OutDataTypeStr=Bus: innerLoopCmdsBus  NonVirtualBus=on
  Bus Selector2 : BusSelector  OutputSignals=pos_vel.z,pos_vel.vy,pos_vel.vx
  Constant : Constant  Value=0  OutDataTypeStr=single
  Constant1 : Constant  Value=UAVSampleTime*4*4  OutDataTypeStr=single
  Mux1 : Mux  Inputs=2
  Saturation : Saturate  UpperLimit=-0.5  LowerLimit=-inf
  Selector : Selector  NumberOfDimensions=2  InputPortWidth=3  IndexOptions=Index vector (dialog),Index vector (dialog)  Indices=3,[1 2]  OutputSizes=1,1
  Sum : Sum
  Transpose : Math  Operator=transpose  SaturateOnIntegerOverflow=on
  InnerLoopCmds1 : Outport  OutDataTypeStr=Bus: innerLoopCmdsBus
  wires:
  Mux1/1 -> Bus Creator1/1  "LAP"
  Bus Selector2/2 -> Atan1/1  "<vy>"
  Bus Selector2/3 -> Atan1/2  "<vx>"
  Atan1/1 -> Bus Creator1/2  "HeadingCmd"
  UAVState1/1 -> Bus Selector2/1
  Bus Creator1/1 -> InnerLoopCmds1/1
  GCSCmds/1 -> Selector/1
  Selector/1 -> Transpose/1
  Transpose/1 -> Mux1/1
  Constant/1 -> Bus Creator1/3  "YawCmd"
  Sum/1 -> Saturation/1
  Bus Selector2/1 -> Sum/2  "<z>"
  Constant1/1 -> Sum/1
  Saturation/1 -> Mux1/2

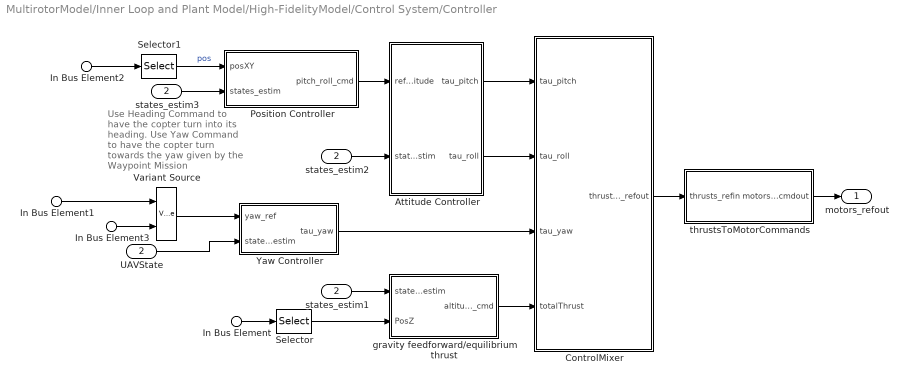
== system MultirotorModel/Inner Loop and Plant Model/High-FidelityModel/Control System/Controller ==
  note: Use Heading Command to have
      | the copter turn into its heading.
      | Use Yaw Command to have the
      | copter turn towards the yaw given
      | by the Waypoint Mission
  In Bus Element2 : Inport  PortName=PositionCmd  Element=LAP
  In Bus Element : Inport  PortName=PositionCmd  Element=LAP
  In Bus Element3 : Inport  PortName=PositionCmd  Element=YawCmd
  In Bus Element1 : Inport  PortName=PositionCmd  Element=HeadingCmd
  UAVState : Inport  Port=2
  Attitude Controller : Subsystem
  ControlMixer : Subsystem
  Position Controller : Subsystem
  Selector : Selector  InputPortWidth=3  IndexOptions=Index vector (dialog)  Indices=3  OutputSizes=1
  Selector1 : Selector  InputPortWidth=3  IndexOptions=Index vector (dialog)  Indices=[1 2]  OutputSizes=1
  Variant Source : VariantSource
  Yaw Controller : Subsystem
  gravity feedforward/equilibrium thrust : Subsystem
  states_estim1 : InportShadow  Port=2
  states_estim2 : InportShadow  Port=2
  states_estim3 : InportShadow  Port=2
  thrustsToMotorCommands : Subsystem
  motors_refout : Outport  VectorParamsAs1DForOutWhenUnconnected=off
  wires:
  Yaw Controller/1(tau_yaw) -> ControlMixer/3(tau_yaw)
  thrustsToMotorCommands/1(motors_cmdout) -> motors_refout/1
  states_estim3/1 -> Position Controller/2(states_estim)
  ControlMixer/1(thrusts_refout) -> thrustsToMotorCommands/1(thrusts_refin)
  gravity feedforward/equilibrium thrust/1(altitude_cmd) -> ControlMixer/4(totalThrust)
  Selector1/1 -> Position Controller/1(posXY)  "pos"
  states_estim1/1 -> gravity feedforward/equilibrium thrust/1(states_estim)
  UAVState/1 -> Yaw Controller/2(states_estim)
  states_estim2/1 -> Attitude Controller/2(states_estim)
  In Bus Element2/1 -> Selector1/1
  In Bus Element/1 -> Selector/1
  Selector/1 -> gravity feedforward/equilibrium thrust/2(PosZ)
  Attitude Controller/1(tau_pitch) -> ControlMixer/1(tau_pitch)
  Attitude Controller/2(tau_roll) -> ControlMixer/2(tau_roll)
  In Bus Element3/1 -> Variant Source/2
  Position Controller/1(pitch_roll_cmd) -> Attitude Controller/1(refAttitude)
  Variant Source/1 -> Yaw Controller/1(yaw_ref)
  In Bus Element1/1 -> Variant Source/1

== system MultirotorModel/Inner Loop and Plant Model/High-FidelityModel/Plant Model/AC model ==
  Actuators : Inport
  Environment : Inport  Port=2
  DCM_be : Inport  Port=3
  V_b : Inport  Port=4  Unit=m/s
  w_b : Inport  Port=5  Unit=rad/s
  Applied Force Calculation : Subsystem
  Bus Selector : BusSelector  OutputSignals=Gravity_ned,AtmosphereBus.air_density
  Drag Calculation : Subsystem
  Gravity Force Calculation : Subsystem
  Motor Forces and Torques : Subsystem
  F_cg : Outport  Unit=N  VectorParamsAs1DForOutWhenUnconnected=off
  M_cg : Outport  Port=2  Unit=N*m  VectorParamsAs1DForOutWhenUnconnected=off
  wires:
  Applied Force Calculation/1(External Forces) -> F_cg/1
  Motor Forces and Torques/2(Motor Torques) -> M_cg/1
  Motor Forces and Torques/1(Motor Forces) -> Applied Force Calculation/3(Motor Forces)
  Bus Selector/1 -> Gravity Force Calculation/2(gravity)  "<Gravity_ned>"
  Gravity Force Calculation/1(gravity force) -> Applied Force Calculation/1(gravity force)
  Environment/1 -> Bus Selector/1
  Bus Selector/2 -> Motor Forces and Torques/2(Density), Drag Calculation/1(Density)  "<air_density>"
  DCM_be/1 -> Gravity Force Calculation/1(DCMbe)
  V_b/1 -> Motor Forces and Torques/1(Vb), Drag Calculation/2(Vb)
  Drag Calculation/1(Drag) -> Applied Force Calculation/2(Aerodynamic Forces)
  Actuators/1 -> Motor Forces and Torques/4(Motor Commands)
  w_b/1 -> Motor Forces and Torques/3(pqr)

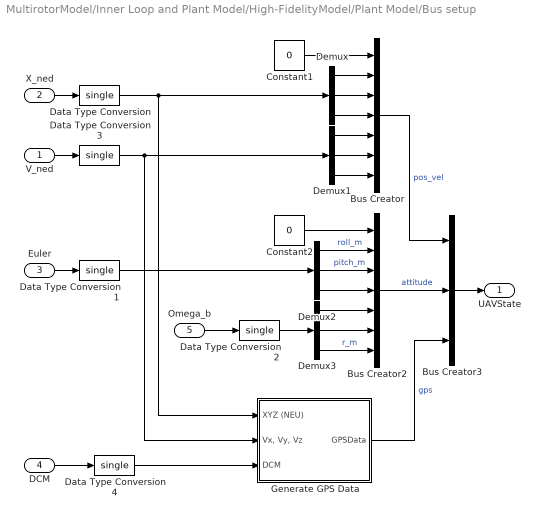
== system MultirotorModel/Inner Loop and Plant Model/High-FidelityModel/Plant Model/Bus setup ==
  V_ned : Inport  Unit=m/second  PortDimensions=3
  X_ned : Inport  Port=2  Unit=m  PortDimensions=3
  Euler : Inport  Port=3  Unit=rad  PortDimensions=3
  DCM : Inport  Port=4
  Omega_b : Inport  Port=5  Unit=rad/s  PortDimensions=3
  Bus Creator : BusCreator  Inputs=7  OutDataTypeStr=Bus: local_position_ned
      settings: InheritFromInputs=off
  Bus Creator2 : BusCreator  Inputs=7  OutDataTypeStr=Bus: attitudeBus
      settings: InheritFromInputs=off
  Bus Creator3 : BusCreator  Inputs=3  OutDataTypeStr=Bus: uavStateBus
      settings: InheritFromInputs=off
  Constant1 : Constant  Value=0  OutDataTypeStr=uint32
  Constant2 : Constant  Value=0  OutDataTypeStr=uint32
  Data Type Conversion{,1..4} (5 alike) : DataTypeConversion  OutDataTypeStr=single
  Demux{,1..3} (4 alike) : Demux  Outputs=3
  Generate GPS Data : Subsystem
  UAVState : Outport  OutDataTypeStr=Bus: uavStateBus
  wires:
  Demux1/3 -> Bus Creator/7
  Bus Creator3/1 -> UAVState/1
  Demux/2 -> Bus Creator/3
  Demux3/2 -> Bus Creator2/6
  Bus Creator2/1 -> Bus Creator3/2  "attitude"
  Demux1/2 -> Bus Creator/6
  Demux3/1 -> Bus Creator2/5
  Demux/1 -> Bus Creator/2
  Euler/1 -> Data Type Conversion1/1
  Demux2/3 -> Bus Creator2/4
  Demux2/1 -> Bus Creator2/2  "roll_m"
  Bus Creator/1 -> Bus Creator3/1  "pos_vel"
  Constant2/1 -> Bus Creator2/1
  Demux2/2 -> Bus Creator2/3  "pitch_m"
  Demux3/3 -> Bus Creator2/7  "r_m"
  Demux1/1 -> Bus Creator/5
  V_ned/1 -> Data Type Conversion3/1
  Omega_b/1 -> Data Type Conversion2/1
  Demux/3 -> Bus Creator/4
  Constant1/1 -> Bus Creator/1
  Generate GPS Data/1(GPSData) -> Bus Creator3/3  "gps"
  X_ned/1 -> Data Type Conversion/1
  Data Type Conversion/1 -> Generate GPS Data/1(XYZ (NEU)), Demux/1
  Data Type Conversion2/1 -> Demux3/1
  Data Type Conversion1/1 -> Demux2/1
  Data Type Conversion3/1 -> Demux1/1, Generate GPS Data/2("Vx, Vy, Vz")
  DCM/1 -> Data Type Conversion4/1
  Data Type Conversion4/1 -> Generate GPS Data/3(DCM)

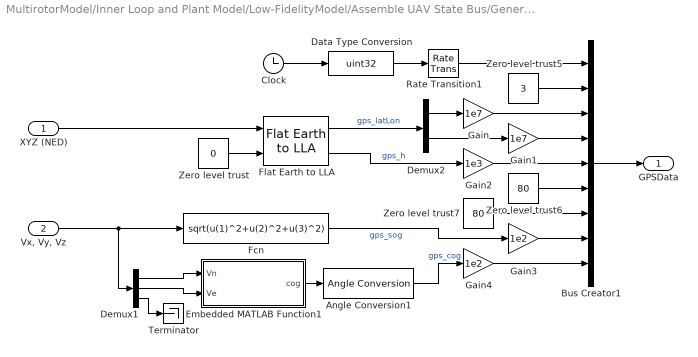
== system MultirotorModel/Inner Loop and Plant Model/Low-FidelityModel/Assemble UAV State Bus/Generate GPS Data ==
  XYZ (NED) : Inport
  "Vx, Vy, Vz" : Inport  Port=2
  Angle Conversion1 : aerolibconvert2/Angle Conversion  IU=rad  OU=deg
  Bus Creator1 : BusCreator  Inputs=9  OutDataTypeStr=Bus: gps_raw_int  NonVirtualBus=on
      settings: InheritFromInputs=off
  Clock : Clock
      settings: AttributesFormatString=Decimation: %<Decimation>
  Data Type Conversion : DataTypeConversion  OutDataTypeStr=uint32
  Demux1 : Demux  Outputs=3
  Demux2 : Demux  Outputs=2
  Embedded MATLAB Function1 : MATLAB Function  TreatAsAtomicUnit=on
  Fcn : Fcn  Expr=sqrt(u(1)^2+u(2)^2+u(3)^2)
  Flat Earth to LLA : aerolibtransform2/Flat Earth to LLA  units=Metric (MKS)  ptype=Earth (WGS84)  F=1/298.257223563  R=6378137  refPosPort=off  LL0=uavIC_latLon  psi=0
  Gain : Gain  Gain=1e7  OutDataTypeStr=int32
  Gain1 : Gain  Gain=1e7  OutDataTypeStr=int32
  Gain2 : Gain  Gain=1e3  OutDataTypeStr=int32
  Gain3 : Gain  Gain=1e2  OutDataTypeStr=uint16
  Gain4 : Gain  Gain=1e2  OutDataTypeStr=uint16
  Rate Transition1 : RateTransition  OutPortSampleTime=0.005
  Terminator : Terminator
  Zero level trust : Constant  Value=0
      settings: AttributesFormatString=%<Value>
  Zero level trust5 : Constant  Value=3  OutDataTypeStr=uint8
      settings: AttributesFormatString=%<Value>
  Zero level trust6 : Constant  Value=80  OutDataTypeStr=uint16
      settings: AttributesFormatString=%<Value>
  Zero level trust7 : Constant  Value=80  OutDataTypeStr=uint16
      settings: AttributesFormatString=%<Value>
  GPSData : Outport  VectorParamsAs1DForOutWhenUnconnected=off
  wires:
  Demux1/3 -> Terminator/1
  Angle Conversion1/1 -> Gain4/1  "gps_cog"
  Embedded MATLAB Function1/1(cog) -> Angle Conversion1/1
  "Vx, Vy, Vz"/1 -> Demux1/1, Fcn/1
  Demux1/2 -> Embedded MATLAB Function1/2(Ve)
  Demux1/1 -> Embedded MATLAB Function1/1(Vn)
  Fcn/1 -> Gain3/1  "gps_sog"
  Flat Earth to LLA/1 -> Demux2/1  "gps_latLon"
  Zero level trust/1 -> Flat Earth to LLA/2
  XYZ (NED)/1 -> Flat Earth to LLA/1
  Clock/1 -> Data Type Conversion/1
  Flat Earth to LLA/2 -> Gain2/1  "gps_h"
  Demux2/1 -> Gain/1
  Demux2/2 -> Gain1/1
  Zero level trust5/1 -> Bus Creator1/2
  Gain1/1 -> Bus Creator1/4
  Zero level trust6/1 -> Bus Creator1/6
  Gain3/1 -> Bus Creator1/8
  Zero level trust7/1 -> Bus Creator1/7
  Gain4/1 -> Bus Creator1/9
  Gain2/1 -> Bus Creator1/5
  Gain/1 -> Bus Creator1/3
  Data Type Conversion/1 -> Rate Transition1/1
  Bus Creator1/1 -> GPSData/1
  Rate Transition1/1 -> Bus Creator1/1

== system MultirotorModel/Inner Loop and Plant Model/Low-FidelityModel/Position and Acceleration Control/Attitude Control ==
  note: Use Heading Command to have
      | the copter turn into its heading.
      | Use Yaw Command to have the
      | copter turn towards the yaw given
      | by the Waypoint Mission
  Accel Cmd : Inport
  QuadRotorState : Inport  Port=2
  PositionCmd : Inport  Port=3
  Bus Creator : BusCreator  Inputs=4  OutDataTypeStr=Bus: uavGuidanceControlBus  NonVirtualBus=on
      settings: InheritFromInputs=off
  Bus Selector : BusSelector  OutputSignals=HeadingCmd,YawCmd
  Bus Selector1 : BusSelector  OutputSignals=EulerZYX
  Multirotor Acceleration Control : MATLAB Function  TreatAsAtomicUnit=on
  Multirotor Thrust Control : MATLAB Function  TreatAsAtomicUnit=on
  P Gain : Gain  Gain=1.1
  Selector1 : Selector  InputPortWidth=3  IndexOptions=Index vector (dialog)  Indices=[1]  OutputSizes=1
  Sum : Sum  Inputs=-+|
  Variant Source : VariantSource
  dT Limit : Saturate  UpperLimit=1.2  LowerLimit=0
      settings: AttributesFormatString=[%<UpperLimit> %<LowerLimit>]
  phi Limit : Saturate  UpperLimit=25*pi/180  LowerLimit=-25*pi/180
      settings: AttributesFormatString=[%<UpperLimit> %<LowerLimit>]
  psi_dot Limit : Saturate  UpperLimit=30*pi/180  LowerLimit=-30*pi/180
      settings: AttributesFormatString=[%<UpperLimit> %<LowerLimit>]
  theta Limit : Saturate  UpperLimit=25*pi/180  LowerLimit=-25*pi/180
      settings: AttributesFormatString=[%<UpperLimit> %<LowerLimit>]
  Control Signal : Outport
  wires:
  Multirotor Thrust Control/1(thrust) -> dT Limit/1  "Thrust"
  QuadRotorState/1 -> Bus Selector1/1
  Multirotor Acceleration Control/1(roll) -> phi Limit/1  "Roll"
  Bus Creator/1 -> Control Signal/1
  dT Limit/1 -> Bus Creator/4  "thrust"
  P Gain/1 -> psi_dot Limit/1  "YawRate"
  Accel Cmd/1 -> Multirotor Thrust Control/1(acc), Multirotor Acceleration Control/1(acc)
  theta Limit/1 -> Bus Creator/2, Multirotor Thrust Control/2(pitch)  "Pitch"
  Sum/1 -> P Gain/1
  Selector1/1 -> Sum/1, Multirotor Acceleration Control/2(yaw)
  psi_dot Limit/1 -> Bus Creator/3  "YawRate"
  Bus Selector/2 -> Variant Source/2  "<YawCmd>"
  phi Limit/1 -> Bus Creator/1, Multirotor Thrust Control/3(roll)  "Roll"
  Variant Source/1 -> Sum/2
  Bus Selector1/1 -> Selector1/1  "<EulerZYX>"
  PositionCmd/1 -> Bus Selector/1
  Multirotor Acceleration Control/2(pitch) -> theta Limit/1  "Pitch"
  Bus Selector/1 -> Variant Source/1  "<HeadingCmd>"
